simulink model "flight_sim"  (R2013b)
settings: Solver=ode45  StartTime=0.0  StopTime=350  RelTol=1e-3
values from neighbouring files (symbols this model uses):
  g = 9.81    [params.m]
  gam_0 = pi/2    (= 1.57079632679)    [params.m]
  gam_in = 0.10    (= 0.1)    [params.m]
  h_0 = 0    [params.m]
  m_dot = 132    [params.m]
  m_zfw = m_pay+m_dry    (= 6360.7)    [params.m]
  R_E = 6371e3    (= 6371000)    [params.m]
  t_turn = 30.0    (= 30)    [params.m]
  v_0 = 0.01    [params.m]
  x_0 = 0    [params.m]
libraries: simulink x2, aerolibanim x1
settings Model: Creator=Talha Israr  LastModifiedBy=Talha Israr

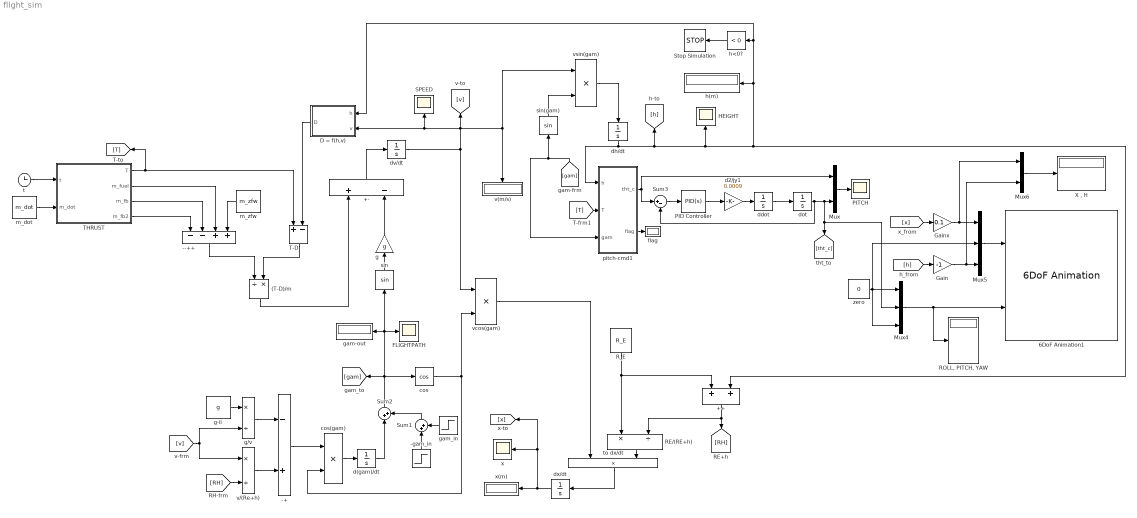
== system flight_sim ==
  (T-D)/m : Product  Inputs=/*
  ++ : Sum
  +- : Sum  Inputs=+-
  -+ : Sum  Inputs=-+
  --++ : Sum  Inputs=--++
  -gam_in : Step  Time=t_turn+1  Before=-gam_in  After=-gam_in  SampleTime=0
  6DoF Animation1 : aerolibanim/6DoF Animation  u1=[-100 10000 -10000 10000 0 10000]  u2=0.3  u3=2000  u4=[100000 100000 -100000]  u5=Fixed position  u6=[-20000 50000 -3500]  u7=10  u8=on
  D = f(h,v) : MATLAB Function  TreatAsAtomicUnit=on
  FLIGHTPATH : Scope
      settings: YMin=-1.5  YMax=1.75  SaveName=ScopeData3  MaxDataPoints=10000
  Gain : Gain  Gain=-1
  Gainx : Gain  Gain=0.1
  HEIGHT : Scope
      settings: YMin=0  YMax=32500  MaxDataPoints=10000
  Mux : Mux  Inputs=2
  Mux4 : Mux  Inputs=3
  Mux5 : Mux  Inputs=3
  Mux6 : Mux  Inputs=2
  PID Controller : simulink/Continuous/PID Controller  Controller=PID  TimeDomain=Continuous-time  SampleTime=1  IntegratorMethod=Forward Euler  FilterMethod=Forward Euler  Form=Parallel  P=0  I=0  D=200/5  N=100  InitialConditionSource=internal  InitialConditionForIntegrator=0  InitialConditionForFilter=0  ExternalReset=none  LimitOutput=off  UpperSaturationLimit=inf  LowerSaturationLimit=-inf  LinearizeAsGain=on  AntiWindupMode=none  Kb=1  TrackingMode=off  Kt=1  PParamMin=[]  PParamMax=[]  IParamMin=[]  IParamMax=[]  DParamMin=[]  DParamMax=[]  NParamMin=[]  NParamMax=[]  KbParamMin=[]  KbParamMax=[]  KtParamMin=[]  KtParamMax=[]  POutMin=[]  POutMax=[]  IOutMin=[]  IOutMax=[]  DOutMin=[]  DOutMax=[]  NOutMin=[]  NOutMax=[]  KbOutMin=[]  KbOutMax=[]  KtOutMin=[]  KtOutMax=[]  IntegratorOutMin=[]  IntegratorOutMax=[]  FilterOutMin=[]  FilterOutMax=[]  SumOutMin=[]  SumOutMax=[]  SumI1OutMin=[]  SumI1OutMax=[]  SumI2OutMin=[]  SumI2OutMax=[]  SumI3OutMin=[]  SumI3OutMax=[]  SumDOutMin=[]  SumDOutMax=[]  SaturationOutMin=[]  SaturationOutMax=[]  IntegratorContinuousStateAttributes=''  IntegratorStateMustResolveToSignalObject=off  IntegratorRTWStateStorageClass=Auto  FilterContinuousStateAttributes=''  FilterStateMustResolveToSignalObject=off  FilterRTWStateStorageClass=Auto
  PITCH : Scope
      settings: YMin=0.25  YMax=3.25  SaveName=ScopeData4  MaxDataPoints=10000
  RE/(RE+h) : Product  Inputs=*/
  "ROLL, PITCH, YAW" : Display
  R_E : Constant  Value=R_E
  SPEED : Scope
      settings: MaxDataPoints=10000
  Stop Simulation : Stop
  Sum1 : Sum  Inputs=|++
  Sum2 : Sum  Inputs=|++
  Sum3 : Sum  Inputs=|+-
  T-D : Sum  Inputs=+-
  THRUST : MATLAB Function  TreatAsAtomicUnit=on
  "X , H" : Display
  cos : Trigonometry  Operator=cos  OutputSignalType=real
  cos(gam) : Product
  d(gam)/dt : Integrator  InitialCondition=gam_0
  d2/jy1 : Gain  Gain=0.0009
  ddot : Integrator
  dh/dt : Integrator  InitialCondition=h_0
  dot : Integrator  InitialCondition=pi/2
  dv/dt : Integrator  InitialCondition=v_0
  dx/dt : Integrator  InitialCondition=x_0
  flag : Display
  g : Gain  Gain=g
  g-ii : Constant  Value=g
  g/v : Product  Inputs=*/
  gam-out : Display
  gam_in : Step  Time=t_turn  Before=gam_in  After=0  SampleTime=0
  h(m) : Display
  h<0? : simulink/Logic and Bit Operations/Compare To Zero  relop=<  OutDataTypeStr=boolean
  m_dot : Constant  Value=m_dot
  m_zfw : Constant  Value=m_zfw
  pitch-cmd1 : MATLAB Function  TreatAsAtomicUnit=on
  sin : Trigonometry
  sin(gam) : Trigonometry
  t : Clock
  to dx/dt : Product
  v(m/s) : Display
  v/(Re+h) : Product  Inputs=*/
  vcos(gam) : Product
  vsin(gam) : Product
  x : Scope
      settings: YMin=0  YMax=85000  SaveName=ScopeData2  MaxDataPoints=10000
  x(m) : Display
  "zero " : Constant  Value=0
  wires:
  t/1 -> THRUST/1(t)
  m_dot/1 -> THRUST/2(m_dot)
  THRUST/1(T) -> T-D/1, [T]
  T-D/1 -> (T-D)/m/2
  (T-D)/m/1 -> +-/1
  dv/dt/1 -> v(m/s)/1, vsin(gam)/1, D = f(h,v)/2(v), SPEED/1, [v], vcos(gam)/1
  vsin(gam)/1 -> dh/dt/1
  D = f(h,v)/1(D) -> T-D/2
  RE/(RE+h)/1 -> to dx/dt/2
  to dx/dt/1 -> dx/dt/1
  ++/1 -> RE/(RE+h)/2, [RH]
  [v] -> g/v/2, v/(Re+h)/1
  [RH] -> v/(Re+h)/2
  g-ii/1 -> g/v/1
  v/(Re+h)/1 -> -+/2
  g/v/1 -> -+/1
  -+/1 -> cos(gam)/1
  cos(gam)/1 -> d(gam)/dt/1
  d(gam)/dt/1 -> Sum2/1
  vcos(gam)/1 -> to dx/dt/1
  Sum2/1 -> [gam], cos/1, FLIGHTPATH/1, gam-out/1, sin/1
  gam_in/1 -> Sum1/2
  -gam_in/1 -> Sum1/1
  Sum1/1 -> Sum2/2
  cos/1 -> cos(gam)/2, vcos(gam)/2
  THRUST/4(m_fb2) -> --++/1
  THRUST/3(m_fb) -> --++/2
  THRUST/2(m_fuel) -> --++/3
  m_zfw/1 -> --++/4
  --++/1 -> (T-D)/m/1
  sin/1 -> g/1
  g/1 -> +-/2
  +-/1 -> dv/dt/1
  R_E/1 -> ++/1, RE/(RE+h)/1
  h<0?/1 -> Stop Simulation/1
  dx/dt/1 -> [x], x/1, x(m)/1
  dh/dt/1 -> pitch-cmd1/1(h), [h], ++/2, h<0?/1, D = f(h,v)/1(h), h(m)/1, HEIGHT/1
  [T] -> pitch-cmd1/2(T)
  pitch-cmd1/2(flag) -> flag/1
  pitch-cmd1/1(tht_c) -> Sum3/1, Mux/1
  Sum3/1 -> PID Controller/1
  ddot/1 -> dot/1
  dot/1 -> Mux4/2, [tht_c], Mux/2, Sum3/2
  Mux/1 -> PITCH/1
  PID Controller/1 -> d2/jy1/1
  d2/jy1/1 -> ddot/1
  sin(gam)/1 -> vsin(gam)/2
  [gam] -> pitch-cmd1/3(gam), sin(gam)/1
  "zero "/1 -> Mux5/2, Mux4/3, Mux4/1
  Mux4/1 -> "ROLL, PITCH, YAW"/1, 6DoF Animation1/2
  Mux5/1 -> 6DoF Animation1/1
  [h] -> Gain/1
  Gain/1 -> Mux6/2, Mux5/3
  [x] -> Gainx/1
  Gainx/1 -> Mux6/1, Mux5/1
  Mux6/1 -> "X , H"/1

== matlab function flight_sim/THRUST ==
  data: T output; m_fuel output; m_fb output; m_fb2 output; t input; m_dot input
function [T,m_fuel,m_fb,m_fb2]= fcn(t,m_dot)
%#codegen
persistent mfb;
persistent mfb2;
if isempty(mfb)
    mfb = 0;
end    
if isempty(mfb2)
    mfb2 = 0;
end  

mfuel = 21491.26;
if mfb<= 0.65*mfuel
    THR = 346961.2;
    mfb = t*m_dot;
else
    THR = 0;
end    

if (125<t) && (t<295)
    THR = -110000;
    mfb2 = (t-125)*(m_dot/3);
end

T = THR;
m_fb = mfb;
m_fb2 = mfb2;
m_fuel = mfuel;

== matlab function flight_sim/D = f(h,v) ==
  data: h input; D output; v input
function D = fcn(h,v)
%#codegen
CD = 0.075;
Di = 1.5;
A = pi*Di^2/4;

if h<=11000
    T = 15.04-0.00649*h;
    p = 101.29*((T+273.1)/288.08)^5.258;
    
elseif (11000<h) && (h <=25000)
    T = -56.46;
    p = 22.65*exp(1.73-0.000157*h);
    
else
    T = -131.21 + 0.00299*h;
    p = 2.488*((T+273.1)/216.6)^-11.388;
end

rho = p/(0.2869*(T+273.1));

Drag = 0.5*rho*v^2*A*CD;

D = Drag;

== matlab function flight_sim/pitch-cmd1 ==
  data: h input; tht_c output; flag output; T input; gam input
function [tht_c, flag] = fcn(h,T,gam)
%#codegen

persistent f

if isempty(f)
    f = 0;
end

if T<=0
    t_c = gam+pi;
    if t_c>pi
        t_c = pi;
    end
    f = 1;
elseif T<=0 && h<1000
    t_c = pi/2;
else
    t_c = gam;
end

flag = f;
tht_c = t_c;
